simulink library "calcAeroLoadsInBdyFrame_cl"  (R2020a)
settings: Solver=VariableStepAuto  StartTime=0.0  StopTime=10.0  RelTol=1e-3
libraries: calcAeroCoeffs_cl x1, calcAoA_Beta_relativeSpeed_ul x1, calc_pqrHat_ul x1, makeBcW_cl x1
settings Model: Creator=Ayaz  LastModifiedBy=Ayaz

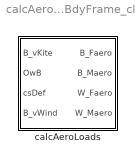
== system calcAeroLoadsInBdyFrame_cl ==
  calcAeroLoads : Subsystem  mask{refArea=3, refSpan=5.5, refChord=0.55, rho=1.225, C_X_AoA_coeffs=[8.32,0], C_X_qHat_coeffs=[4.41,-.6], C_X_dElev_coeffs=[0.11,-.01], C_X_0=0.46, C_Y_Beta_coeffs=-0.19, C_Y_pHat_coeffs=-0.1, C_Y_rHat_coeffs=[0.14,0.17], C_Y_dAil_coeffs=-0.05, C_Y_dRud_coeffs=0.1, C_Z_AoA_coeffs=[10.2,1.23,0], C_Z_qHat_coeffs=[6.15,0.13,-7.56], C_Z_dElev_coeffs=[0.29,0,-0.32], C_Z_0=-5.4, C_l_Beta_coeffs=-0.06, C_l_pHat_coeffs=-0.56, C_l_rHat_coeffs=[0.65,0.18], C_l_dAil_coeffs=[0.04,-0.25], C_l_dRud_coeffs=0, C_m_AoA_coeffs=[0.21,0], C_m_qHat_coeffs=[5.29,0,-11.30], C_m_dElev_coeffs=-1.02, C_m_0=-0.32, C_n_Beta_coeffs=[-0.09,0.06], C_n_pHat_coeffs=[-0.91,-0.06], C_n_rHat_coeffs=-0.05, C_n_dAil_coeffs=[-0.12,0.02], C_n_dRud_coeffs=-.04}
      mask prompts: refArea "Reference wing area [m^2]"; refSpan "Reference wing span [m]"; refChord "Reference wing chord [m]"; rho "Air density [kg/m^3]"; C_X_AoA_coeffs "C_X_AoA polynomial coefficients (c0,c1,c2):"; C_X_qHat_coeffs "C_X_qHat polynomial coefficients (c0,c1,c2):"; C_X_dElev_coeffs "C_X_dElev polynomial coefficients (c0,c1,c2):"; C_X_0 "C_X_0 value"; C_Y_Beta_coeffs "C_Y_Beta polynomial coefficients (c0,c1,c2):"; C_Y_pHat_coeffs "C_Y_pHat polynomial coefficients (c0,c1,c2):"; C_Y_rHat_coeffs "C_Y_rHat polynomial coefficients (c0,c1,c2):"; C_Y_dAil_coeffs "C_Y_dAil polynomial coefficients (c0,c1,c2):"; C_Y_dRud_coeffs "C_Y_dRud polynomial coefficients (c0,c1,c2):"; C_Z_AoA_coeffs "C_Z_AoA polynomial coefficients (c0,c1,c2):"; C_Z_qHat_coeffs "C_Z_qHat polynomial coefficients (c0,c1,c2):"; C_Z_dElev_coeffs "C_Z_dElev polynomial coefficients (c0,c1,c2):"; C_Z_0 "C_Z_0 value"; C_l_Beta_coeffs "C_l_Beta polynomial coefficients (c0,c1,c2):"; C_l_pHat_coeffs "C_l_pHat polynomial coefficients (c0,c1,c2):"; C_l_rHat_coeffs "C_l_rHat polynomial coefficients (c0,c1,c2):"; C_l_dAil_coeffs "C_l_dAil polynomial coefficients (c0,c1,c2):"; C_l_dRud_coeffs "C_l_dRud polynomial coefficients (c0,c1,c2):"; C_m_AoA_coeffs "C_m_AoA polynomial coefficients (c0,c1,c2):"; C_m_qHat_coeffs "C_m_qHat polynomial coefficients (c0,c1,c2):"; C_m_dElev_coeffs "C_m_dElev polynomial coefficients (c0,c1,c2):"; C_m_0 "C_m_0 value"; C_n_Beta_coeffs "C_n_Beta polynomial coefficients (c0,c1,c2):"; C_n_pHat_coeffs "C_n_pHat polynomial coefficients (c0,c1,c2):"; C_n_rHat_coeffs "C_n_rHat polynomial coefficients (c0,c1,c2):"; C_n_dAil_coeffs "C_n_dAil polynomial coefficients (c0,c1,c2):"; C_n_dRud_coeffs "C_n_dRud polynomial coefficients (c0,c1,c2):"
      mask TypeOptions refArea: Constant/Value
      mask TypeOptions refSpan: Constant1/Value | calc_pqrHat/refSpan
      mask TypeOptions refChord: calc_pqrHat/refChord | Constant2/Value
      mask TypeOptions rho: Constant3/Value
      mask TypeOptions C_X_AoA_coeffs: calcAeroCoeffs/C_X_AoA_coeffs
      mask TypeOptions C_X_qHat_coeffs: calcAeroCoeffs/C_X_qHat_coeffs
      mask TypeOptions C_X_dElev_coeffs: calcAeroCoeffs/C_X_dElev_coeffs
      mask TypeOptions C_X_0: calcAeroCoeffs/C_X_0
      mask TypeOptions C_Y_Beta_coeffs: calcAeroCoeffs/C_Y_Beta_coeffs
      mask TypeOptions C_Y_pHat_coeffs: calcAeroCoeffs/C_Y_pHat_coeffs
      mask TypeOptions C_Y_rHat_coeffs: calcAeroCoeffs/C_Y_rHat_coeffs
      mask TypeOptions C_Y_dAil_coeffs: calcAeroCoeffs/C_Y_dAil_coeffs
      mask TypeOptions C_Y_dRud_coeffs: calcAeroCoeffs/C_Y_dRud_coeffs
      mask TypeOptions C_Z_AoA_coeffs: calcAeroCoeffs/C_Z_AoA_coeffs
      mask TypeOptions C_Z_qHat_coeffs: calcAeroCoeffs/C_Z_qHat_coeffs
      mask TypeOptions C_Z_dElev_coeffs: calcAeroCoeffs/C_Z_dElev_coeffs
      mask TypeOptions C_Z_0: calcAeroCoeffs/C_Z_0
      mask TypeOptions C_l_Beta_coeffs: calcAeroCoeffs/C_l_Beta_coeffs
      mask TypeOptions C_l_pHat_coeffs: calcAeroCoeffs/C_l_pHat_coeffs
      mask TypeOptions C_l_rHat_coeffs: calcAeroCoeffs/C_l_rHat_coeffs
      mask TypeOptions C_l_dAil_coeffs: calcAeroCoeffs/C_l_dAil_coeffs
      mask TypeOptions C_l_dRud_coeffs: calcAeroCoeffs/C_l_dRud_coeffs
      mask TypeOptions C_m_AoA_coeffs: calcAeroCoeffs/C_m_AoA_coeffs
      mask TypeOptions C_m_qHat_coeffs: calcAeroCoeffs/C_m_qHat_coeffs
      mask TypeOptions C_m_dElev_coeffs: calcAeroCoeffs/C_m_dElev_coeffs
      mask TypeOptions C_m_0: calcAeroCoeffs/C_m_0
      mask TypeOptions C_n_Beta_coeffs: calcAeroCoeffs/C_n_Beta_coeffs
      mask TypeOptions C_n_pHat_coeffs: calcAeroCoeffs/C_n_pHat_coeffs
      mask TypeOptions C_n_rHat_coeffs: calcAeroCoeffs/C_n_rHat_coeffs
      mask TypeOptions C_n_dAil_coeffs: calcAeroCoeffs/C_n_dAil_coeffs
      mask TypeOptions C_n_dRud_coeffs: calcAeroCoeffs/C_n_dRud_coeffs
      mask DialogControl Container4 Prompt: Kite and envrionment parameters
      mask DialogControl Container5 Prompt: Aero-coefficient parameters
      mask DialogControl Container6 Prompt: CX
      mask DialogControl Container7 Prompt: CY
      mask DialogControl Container8 Prompt: CZ
      mask DialogControl Container9 Prompt: Cl
      mask DialogControl Container10 Prompt: Cm
      mask DialogControl Container11 Prompt: Cn

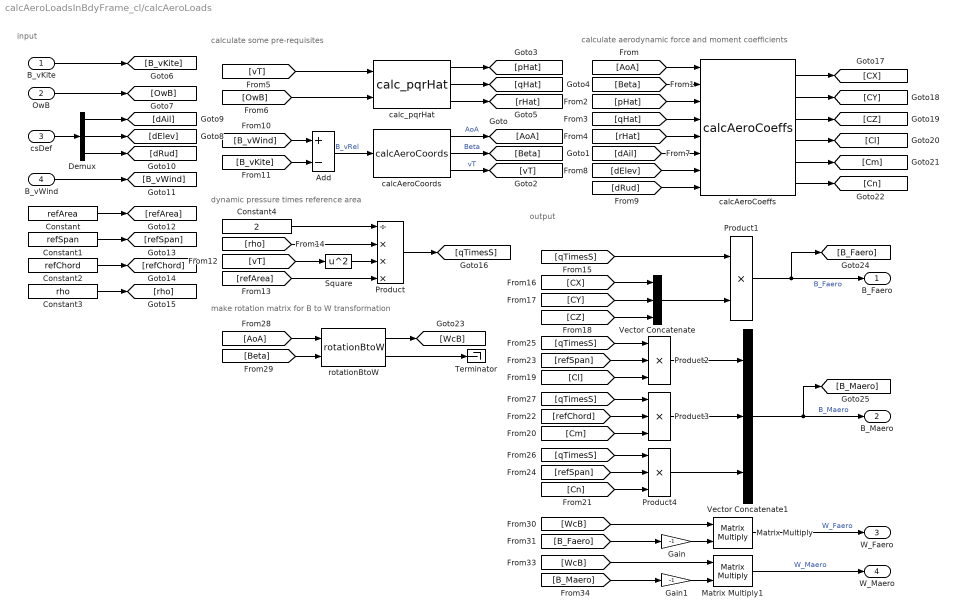
== system calcAeroLoadsInBdyFrame_cl/calcAeroLoads ==
  note: make rotation matrix for B to W transformation
  note: output
  note: calculate aerodynamic force and moment coefficients
  note: dynamic pressure times reference area
  note: calculate some pre-requisites
  note: input
  B_vKite : Inport
  OwB : Inport  Port=2
  csDef : Inport  Port=3
  B_vWind : Inport  Port=4
  Add : Sum  Inputs=+-
  Constant : Constant  Value=refArea
  Constant1 : Constant  Value=refSpan
  Constant2 : Constant  Value=refChord
  Constant3 : Constant  Value=rho
  Constant4 : Constant  Value=2
  Demux : Demux  Outputs=3
  Gain : Gain  Gain=-1
  Gain1 : Gain  Gain=-1
  Matrix Multiply : Product  Multiplication=Matrix(*)
  Matrix Multiply1 : Product  Multiplication=Matrix(*)
  Product : Product  Inputs=/***
  Product1 : Product
  Product2 : Product  Inputs=3
  Product3 : Product  Inputs=3
  Product4 : Product  Inputs=3
  Square : Math  Operator=square  SaturateOnIntegerOverflow=on
  Terminator : Terminator
  Vector Concatenate : Concatenate  NumInputs=3
  Vector Concatenate1 : Concatenate  NumInputs=3
  calcAeroCoeffs : calcAeroCoeffs_cl/calcAeroCoeffs  C_X_AoA_coeffs=C_X_AoA_coeffs  C_X_qHat_coeffs=C_X_qHat_coeffs  C_X_dElev_coeffs=C_X_dElev_coeffs  C_X_0=C_X_0  C_Y_Beta_coeffs=C_Y_Beta_coeffs  C_Y_pHat_coeffs=C_Y_pHat_coeffs  C_Y_rHat_coeffs=C_Y_rHat_coeffs  C_Y_dAil_coeffs=C_Y_dAil_coeffs  C_Y_dRud_coeffs=C_Y_dRud_coeffs  C_Z_AoA_coeffs=C_Z_AoA_coeffs  C_Z_qHat_coeffs=C_Z_qHat_coeffs  C_Z_dElev_coeffs=C_Z_dElev_coeffs  C_Z_0=C_Z_0  C_l_Beta_coeffs=C_l_Beta_coeffs  C_l_pHat_coeffs=C_l_pHat_coeffs  C_l_rHat_coeffs=C_l_rHat_coeffs  C_l_dAil_coeffs=C_l_dAil_coeffs  C_l_dRud_coeffs=C_l_dRud_coeffs  C_m_AoA_coeffs=C_m_AoA_coeffs  C_m_qHat_coeffs=C_m_qHat_coeffs  C_m_dElev_coeffs=C_m_dElev_coeffs  C_m_0=C_m_0  C_n_Beta_coeffs=C_n_Beta_coeffs  C_n_pHat_coeffs=C_n_pHat_coeffs  C_n_rHat_coeffs=C_n_rHat_coeffs  C_n_dAil_coeffs=C_n_dAil_coeffs  C_n_dRud_coeffs=C_n_dRud_coeffs
  calcAeroCoords : calcAoA_Beta_relativeSpeed_ul/calcAeroCoords  SystemSampleTime=-1  Latency=0  AutoFrameSizeCalculation=off
  calc_pqrHat : calc_pqrHat_ul/calc_pqrHat  refSpan=refSpan  refChord=refChord
  rotationBtoW : makeBcW_cl/rotationBtoW  SystemSampleTime=-1  Latency=0  AutoFrameSizeCalculation=off
  B_Faero : Outport  PortDimensions=[3,1]
  B_Maero : Outport  Port=2  PortDimensions=[3,1]
  W_Faero : Outport  Port=3  PortDimensions=[3,1]
  W_Maero : Outport  Port=4  PortDimensions=[3,1]
  wires:
  calcAeroCoords/2 -> [Beta]  "Beta"
  [AoA] -> calcAeroCoeffs/1
  [qHat] -> calcAeroCoeffs/4
  calcAeroCoords/3 -> [vT]  "vT"
  calc_pqrHat/1 -> [pHat]
  [rHat] -> calcAeroCoeffs/5
  [pHat] -> calcAeroCoeffs/3
  calc_pqrHat/2 -> [qHat]
  [Beta] -> calcAeroCoeffs/2
  calcAeroCoords/1 -> [AoA]  "AoA"
  [vT] -> calc_pqrHat/1
  calc_pqrHat/3 -> [rHat]
  B_vKite/1 -> [B_vKite]
  OwB/1 -> [OwB]
  [OwB] -> calc_pqrHat/2
  csDef/1 -> Demux/1
  Demux/2 -> [dElev]
  Demux/1 -> [dAil]
  Demux/3 -> [dRud]
  [dAil] -> calcAeroCoeffs/6
  [dElev] -> calcAeroCoeffs/7
  [dRud] -> calcAeroCoeffs/8
  B_vWind/1 -> [B_vWind]
  Add/1 -> calcAeroCoords/1  "B_vRel"
  [B_vWind] -> Add/1
  [B_vKite] -> Add/2
  Constant/1 -> [refArea]
  Constant1/1 -> [refSpan]
  Constant2/1 -> [refChord]
  Constant3/1 -> [rho]
  [vT] -> Square/1
  Constant4/1 -> Product/1
  Square/1 -> Product/3
  [rho] -> Product/2
  [refArea] -> Product/4
  Product/1 -> [qTimesS]
  calcAeroCoeffs/1 -> [CX]
  calcAeroCoeffs/2 -> [CY]
  calcAeroCoeffs/3 -> [CZ]
  calcAeroCoeffs/4 -> [Cl]
  calcAeroCoeffs/5 -> [Cm]
  calcAeroCoeffs/6 -> [Cn]
  [CY] -> Vector Concatenate/2
  [CZ] -> Vector Concatenate/3
  [qTimesS] -> Product1/1
  Product1/1 -> B_Faero/1, [B_Faero]  "B_Faero"
  [qTimesS] -> Product2/1
  [refSpan] -> Product2/2
  [Cl] -> Product2/3
  [qTimesS] -> Product3/1
  [refChord] -> Product3/2
  [qTimesS] -> Product4/1
  [refSpan] -> Product4/2
  [Cn] -> Product4/3
  Vector Concatenate1/1 -> [B_Maero], B_Maero/1  "B_Maero"
  [AoA] -> rotationBtoW/1
  [Beta] -> rotationBtoW/2
  rotationBtoW/1 -> [WcB]
  rotationBtoW/2 -> Terminator/1
  [WcB] -> Matrix Multiply/1
  [B_Faero] -> Gain/1
  [B_Maero] -> Gain1/1
  [WcB] -> Matrix Multiply1/1
  Matrix Multiply1/1 -> W_Maero/1  "W_Maero"
  Matrix Multiply/1 -> W_Faero/1  "W_Faero"
  Gain/1 -> Matrix Multiply/2
  Gain1/1 -> Matrix Multiply1/2
  [CX] -> Vector Concatenate/1
  [Cm] -> Product3/3
  Vector Concatenate/1 -> Product1/2
  Product2/1 -> Vector Concatenate1/1
  Product3/1 -> Vector Concatenate1/2
  Product4/1 -> Vector Concatenate1/3
